simulink model "first_gear_model"  (R2020b)
settings: Solver=VariableStepAuto  StartTime=0.0  StopTime=5  RelTol=1e-3
libraries: slctrlblks x1
settings Model: Creator=morro  LastModifiedBy=morro

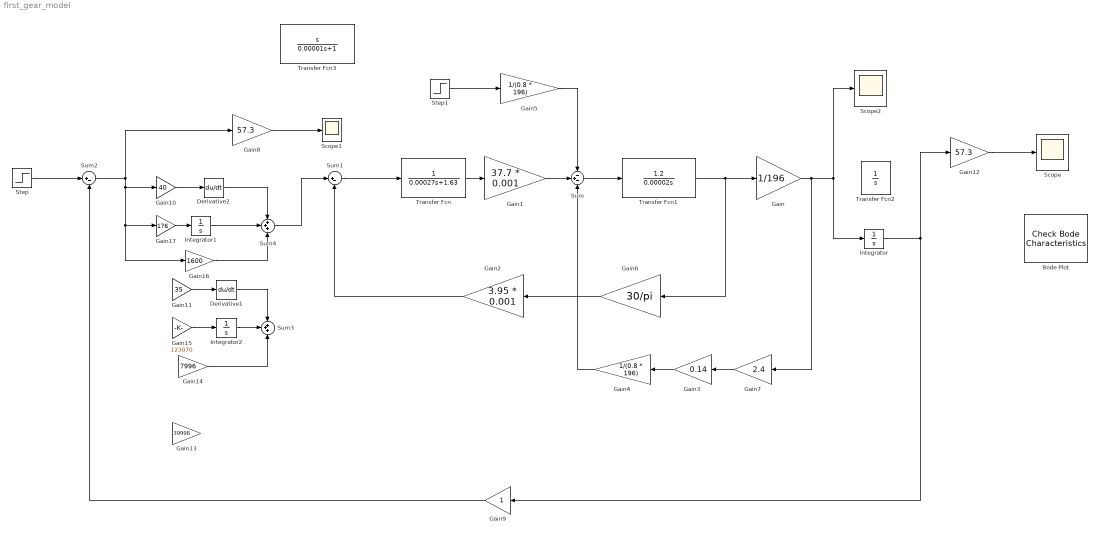
== system first_gear_model ==
  Bode Plot : slctrlblks/Model Verification/Check Bode  Characteristics  InstantiateOnLoad=on  SaveOperatingPoints=off  LinearizationIOs={'/Step', 1, 'in', 'on', '';'/Integrator', 1, 'out', 'on', ''}  LinearizeAt=SnapshotTimes  SnapshotTimes=[0]  TriggerType=rising  SampleTime=auto  RateConversionMethod=zoh  PreWarpFreq=10  UseExactDelayModel=off  UseFullBlockNameLabels=off  UseBusSignalLabels=off  enabled=on  stopWhenAssertionFail=off  export=off  ViewDlgPos=[100 200 510 390]  OpenViewOnLoad=off  LaunchViewOnOpen=off  FrequencyUnits=rad/s  MagnitudeUnits=dB  PhaseUnits=deg  TimeUnits=seconds  EnableUpperBound=off  UpperBoundFrequencies=[]  UpperBoundMagnitudes=[]  EnableLowerBound=off  LowerBoundFrequencies=[]  LowerBoundMagnitudes=[]
  Derivative1 : Derivative
  Derivative2 : Derivative
  Gain : Gain  Gain=1/196
  Gain1 : Gain  Gain=37.7 * 0.001
  Gain10 : Gain  Gain=40
  Gain11 : Gain  Gain=35
  Gain12 : Gain  Gain=57.3
  Gain13 : Gain  Gain=39998
  Gain14 : Gain  Gain=7996
  Gain15 : Gain  Gain=123070
  Gain16 : Gain  Gain=1600
  Gain17 : Gain  Gain=176
  Gain2 : Gain  Gain=3.95 * 0.001
  Gain3 : Gain  Gain=0.14
  Gain4 : Gain  Gain=1/(0.8 * 196)
  Gain5 : Gain  Gain=1/(0.8 * 196)
  Gain6 : Gain  Gain=30/pi
  Gain7 : Gain  Gain=2.4
  Gain8 : Gain  Gain=57.3
  Gain9 : Gain
  Integrator : Integrator  InitialCondition=1e-7
  Integrator1 : Integrator  InitialCondition=1e-7
  Integrator2 : Integrator  InitialCondition=1e-7
  Scope : Scope
  Scope1 : Scope
  Scope2 : Scope
  Step : Step  After=10/57.3  SampleTime=0
  Step1 : Step  Time=1.5  After=9  SampleTime=0
  Sum : Sum  Inputs=-+-
  Sum1 : Sum  Inputs=|+-
  Sum2 : Sum  Inputs=|+-
  Sum3 : Sum  Inputs=+++
  Sum4 : Sum  Inputs=+++
  Transfer Fcn : TransferFcn  Denominator=[0.00027 1.63]
  Transfer Fcn1 : TransferFcn  Numerator=[1.2]  Denominator=[0.00002 0]
  Transfer Fcn2 : TransferFcn  Denominator=[1 0]
  Transfer Fcn3 : TransferFcn  Numerator=[1 0]  Denominator=[0.00001 1]
  wires:
  Transfer Fcn/1 -> Gain1/1
  Sum/1 -> Transfer Fcn1/1
  Gain2/1 -> Sum1/2
  Gain3/1 -> Gain4/1
  Gain1/1 -> Sum/2
  Gain4/1 -> Sum/3
  Gain5/1 -> Sum/1
  Step1/1 -> Gain5/1
  Gain6/1 -> Gain2/1
  Gain/1 -> Gain7/1, Integrator/1, Scope2/1
  Transfer Fcn1/1 -> Gain6/1, Gain/1
  Gain8/1 -> Scope1/1
  Gain9/1 -> Sum2/2
  Step/1 -> Sum2/1
  Gain16/1 -> Sum4/3
  Gain12/1 -> Scope/1
  Integrator/1 -> Gain9/1, Gain12/1
  Gain17/1 -> Integrator1/1
  Integrator1/1 -> Sum4/2
  Sum1/1 -> Transfer Fcn/1
  Gain7/1 -> Gain3/1
  Integrator2/1 -> Sum3/2
  Gain15/1 -> Integrator2/1
  Derivative1/1 -> Sum3/1
  Gain14/1 -> Sum3/3
  Gain11/1 -> Derivative1/1
  Sum2/1 -> Gain10/1, Gain17/1, Gain16/1, Gain8/1
  Sum4/1 -> Sum1/1
  Gain10/1 -> Derivative2/1
  Derivative2/1 -> Sum4/1
